simulink model "EHB_MOTOR0313"  (R2022a)
settings: Solver=FixedStepAuto  StartTime=0.0  StopTime=10  FixedStep=0.0001  RelTol=1e-3  EnableMultiTasking=on
undefined symbols (not defined in the file): Cos_Table, Cos_Table1, Sin_BreakPoint, Sin_BreakPoint1, Sin_Table, Sin_Table1
libraries: simulink x7
(part 1 of 2)
settings Model: Creator=dell  LastModifiedBy=12399
settings SolverCC: AlgebraicLoopSolver=TrustRegion  PositivePriorityOrder=on  AutoInsertRateTranBlk=on
settings DataIOCC: LimitDataPoints=on  SaveFormat=Structure  SignalLoggingSaveFormat=ModelDataLogs  ReturnWorkspaceOutputs=off
settings OptimizationCC: DefaultParameterBehavior=Inlined  UseDivisionForNetSlopeComputation=on  InlineInvariantSignals=on  ExpressionDepthLimit=2147483647  ZeroExternalMemoryAtStartup=off  NoFixptDivByZeroProtection=on  EfficientFloat2IntCast=on  LifeSpan=1  MaxStackSize=64  EfficientTunableParamExpr=on
settings DebuggingCC: CheckSSInitialOutputMsg=off  UnderspecifiedInitializationDetection=Classic  MergeDetectMultiDrivingBlocksExec=none  SignalResolutionControl=TryResolveAll  SolverPrmCheckMsg=warning  ParameterOverflowMsg=none  ParameterPrecisionLossMsg=none  FcnCallInpInsideContextMsg=warning  UnconnectedInputMsg=warning  UnconnectedOutputMsg=warning  UnconnectedLineMsg=warning  AssertControl=EnableAll  StateNameClashWarn=warning  SFUnexpectedBacktrackingDiag=warning  SFNoUnconditionalDefaultTransitionDiag=warning  SFExecutionAtInitializationDiag=none  SFMachineParentedDataDiag=warning  ArithmeticOperatorsInVariantConditions=warning
settings HardwareCC: ProdBitPerPointer=32  ProdBitPerSizeT=32  ProdBitPerPtrDiffT=32  ProdLargestAtomicInteger=Integer  ProdLargestAtomicFloat=None  ProdIntDivRoundTo=Undefined  ProdEndianess=Unspecified  ProdWordSize=32  ProdHWDeviceType=Generic->32-bit Embedded Processor  TargetBitPerPointer=64  TargetBitPerSizeT=64  TargetBitPerPtrDiffT=64  TargetLargestAtomicInteger=Integer  TargetLongLongMode=on  TargetIntDivRoundTo=Zero  TargetEndianess=LittleEndian  TargetWordSize=64  TargetHWDeviceType=MATLAB Host  ProdEqTarget=off
settings ModelReferenceCC: UpdateModelReferenceTargets=IfOutOfDate  PropagateSignalLabelsOutOfModel=off
settings SFSimCC: SimUseLocalCustomCode=off  MATLABDynamicMemAlloc=off  CustomCodeUndefinedFunction=UseInterfaceOnly
settings SFSimCC: SimCustomHeaderCode=|
  | #define MCU_IDLE_ST     0
  | #define MCU_INIT_ST     1
  | #define MCU_START_ST    2
  | #define MCU_RUN_ST      3
  | #define MCU_FAULT_ST    4
  | #define MCU_WAIT_ST     5
  | 
  | // MCU_IDLE_ST = 0;
  | // MCU_INIT_ST = 1;
  | // MCU_START_ST = 2;
  | // MCU_RUN_ST = 3;
  | // MCU_FAULT_ST = 4;
  | // MCU_WAIT_ST = 5;
settings RTWCC: SystemTargetFile=ert.tlc  TemplateMakefile=ert_default_tmf  RTWUseLocalCustomCode=off  RTWUseSimCustomCode=on  IncludeHyperlinkInReport=on
settings RTWCC: CustomHeaderCode=|
  | #define MCU_IDLE_ST     0
  | #define MCU_INIT_ST     1
  | #define MCU_START_ST    2
  | #define MCU_RUN_ST      3
  | #define MCU_FAULT_ST    4
  | #define MCU_WAIT_ST     5
  | 
  | // MCU_IDLE_ST = 0;
  | // MCU_INIT_ST = 1;
  | // MCU_START_ST = 2;
  | // MCU_RUN_ST = 3;
  | // MCU_FAULT_ST = 4;
  | // MCU_WAIT_ST = 5;
settings CodeAppCC: GenerateComments=off  IgnoreCustomStorageClasses=off  CustomSymbolStrType=$N$R$M  SimulinkBlockComments=off  MATLABSourceComments=on  InternalIdentifier=Classic
settings ERTTargetCC: MultiwordLength=2048  IncludeFileDelimiter=UseQuote  SupportContinuousTime=on  InlinedParameterPlacement=NonHierarchical  ERTCustomFileTemplate=example_file_process.tlc  GlobalDataDefinition=InSeparateSourceFile  DataDefinitionFile=EHB_MOTOR_data.c  GlobalDataReference=InSeparateHeaderFile  ERTFilePackagingFormat=CompactWithDataFile  DataReferenceFile=EHB_MOTOR.h  ConvertIfToSwitch=off  SuppressUnreachableDefaultCases=off  IndentStyle=Allman  IndentSize=4  MemSecPackage=mpt
settings ConfigComp: CovMetricSettings=dw  CovSaveCumulativeToWorkspaceVar=on  CovSaveSingleToWorkspaceVar=on  CovExternalEMLEnable=off  CovSFcnEnable=off
settings SimscapeCC: SimscapeNormalizeSystem=off
settings ConfigurationSet: Description=SimMechanics 2G

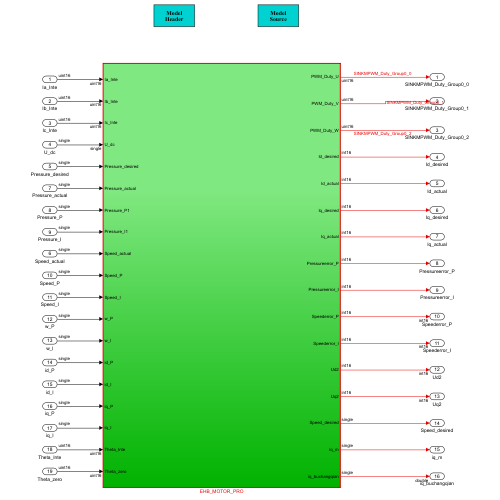
[thumbnail: Simulink's stored preview of the top-level diagram]
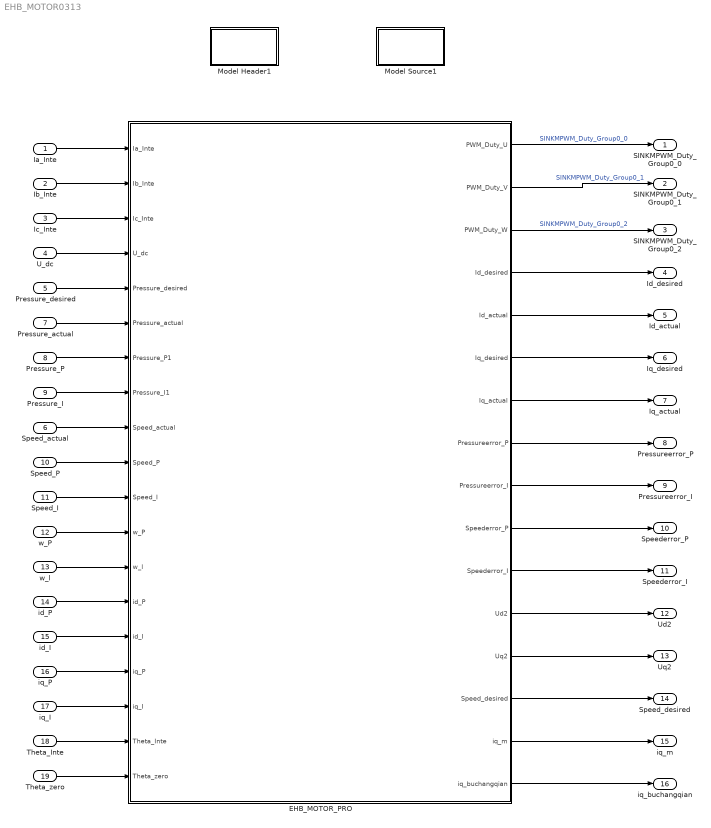
== system EHB_MOTOR0313 ==
  Ia_Inte : Inport  OutDataTypeStr=uint16
  Ib_Inte : Inport  Port=2  OutDataTypeStr=uint16
  Ic_Inte : Inport  Port=3  OutDataTypeStr=uint16
  U_dc : Inport  Port=4  OutDataTypeStr=single
  Pressure_desired : Inport  Port=5  OutDataTypeStr=single
  Speed_actual : Inport  Port=6  OutDataTypeStr=single
  Pressure_actual : Inport  Port=7  OutDataTypeStr=single
  Pressure_P : Inport  Port=8  OutDataTypeStr=single
  Pressure_I : Inport  Port=9  OutDataTypeStr=single
  Speed_P : Inport  Port=10  OutDataTypeStr=single
  Speed_I : Inport  Port=11  OutDataTypeStr=single
  w_P : Inport  Port=12  OutDataTypeStr=single
  w_l : Inport  Port=13  OutDataTypeStr=single
  id_P : Inport  Port=14  OutDataTypeStr=single
  id_I : Inport  Port=15  OutDataTypeStr=single
  iq_P : Inport  Port=16  OutDataTypeStr=single
  iq_I : Inport  Port=17  OutDataTypeStr=single
  Theta_Inte : Inport  Port=18  OutDataTypeStr=uint16
  Theta_zero : Inport  Port=19  OutDataTypeStr=uint16
  EHB_MOTOR_PRO : Subsystem  TreatAsAtomicUnit=on  RTWFcnName=isr_can_rx
      settings: MinAlgLoopOccurrences=on
  Model Header1 : Subsystem  mask(Model Header){ShowInLibBrowser=0}
      mask prompts: ShowInLibBrowser "Simulink:masks:CustCodeMaskParam1_MP"
      settings: CopyFcn=cccopyfcn(gcb)  OpenFcn=ccopenfcn('Model Header')
      mask Help: eval('feval(''rtwprivate'',''rtwhelpview'',''rtw_model_header_block'')');
      mask Display: disp('Model\nHeader');
  Model Source1 : Subsystem  mask(Model Source){ShowInLibBrowser=0}
      mask prompts: ShowInLibBrowser "Simulink:masks:CustCodeMaskParam1_MP"
      settings: CopyFcn=cccopyfcn(gcb)  OpenFcn=ccopenfcn('Model Source')
      mask Help: eval('feval(''rtwprivate'',''rtwhelpview'',''rtw_model_source_block'')');
      mask Display: disp('Model\nSource');
  SINKMPWM_Duty_Group0_0 : Outport  VectorParamsAs1DForOutWhenUnconnected=off
  SINKMPWM_Duty_Group0_1 : Outport  Port=2  VectorParamsAs1DForOutWhenUnconnected=off
  SINKMPWM_Duty_Group0_2 : Outport  Port=3  VectorParamsAs1DForOutWhenUnconnected=off
  Id_desired : Outport  Port=4  VectorParamsAs1DForOutWhenUnconnected=off
  Id_actual : Outport  Port=5  VectorParamsAs1DForOutWhenUnconnected=off
  Iq_desired : Outport  Port=6  VectorParamsAs1DForOutWhenUnconnected=off
  Iq_actual : Outport  Port=7  VectorParamsAs1DForOutWhenUnconnected=off
  Pressureerror_P : Outport  Port=8  VectorParamsAs1DForOutWhenUnconnected=off
  Pressureerror_I : Outport  Port=9  VectorParamsAs1DForOutWhenUnconnected=off
  Speederror_P : Outport  Port=10  OutDataTypeStr=int16  VectorParamsAs1DForOutWhenUnconnected=off
  Speederror_I : Outport  Port=11  OutDataTypeStr=int16  VectorParamsAs1DForOutWhenUnconnected=off
  Ud2 : Outport  Port=12  OutDataTypeStr=int16  VectorParamsAs1DForOutWhenUnconnected=off
  Uq2 : Outport  Port=13  OutDataTypeStr=int16  VectorParamsAs1DForOutWhenUnconnected=off
  Speed_desired : Outport  Port=14
  iq_m : Outport  Port=15
  iq_buchangqian : Outport  Port=16
  wires:
  EHB_MOTOR_PRO/1(PWM_Duty_U) -> SINKMPWM_Duty_Group0_0/1  "SINKMPWM_Duty_Group0_0"
  EHB_MOTOR_PRO/2(PWM_Duty_V) -> SINKMPWM_Duty_Group0_1/1  "SINKMPWM_Duty_Group0_1"
  EHB_MOTOR_PRO/3(PWM_Duty_W) -> SINKMPWM_Duty_Group0_2/1  "SINKMPWM_Duty_Group0_2"
  Theta_Inte/1 -> EHB_MOTOR_PRO/18(Theta_Inte)
  Ia_Inte/1 -> EHB_MOTOR_PRO/1(Ia_Inte)
  U_dc/1 -> EHB_MOTOR_PRO/4(U_dc)
  Ib_Inte/1 -> EHB_MOTOR_PRO/2(Ib_Inte)
  id_P/1 -> EHB_MOTOR_PRO/14(id_P)
  id_I/1 -> EHB_MOTOR_PRO/15(id_I)
  iq_P/1 -> EHB_MOTOR_PRO/16(iq_P)
  iq_I/1 -> EHB_MOTOR_PRO/17(iq_I)
  Theta_zero/1 -> EHB_MOTOR_PRO/19(Theta_zero)
  Pressure_desired/1 -> EHB_MOTOR_PRO/5(Pressure_desired)
  Speed_actual/1 -> EHB_MOTOR_PRO/9(Speed_actual)
  Speed_P/1 -> EHB_MOTOR_PRO/10(Speed_P)
  Speed_I/1 -> EHB_MOTOR_PRO/11(Speed_I)
  EHB_MOTOR_PRO/5(Id_actual) -> Id_actual/1
  EHB_MOTOR_PRO/6(Iq_desired) -> Iq_desired/1
  EHB_MOTOR_PRO/7(Iq_actual) -> Iq_actual/1
  w_l/1 -> EHB_MOTOR_PRO/13(w_l)
  EHB_MOTOR_PRO/10(Speederror_P) -> Speederror_P/1
  EHB_MOTOR_PRO/11(Speederror_I) -> Speederror_I/1
  EHB_MOTOR_PRO/4(Id_desired) -> Id_desired/1
  Ic_Inte/1 -> EHB_MOTOR_PRO/3(Ic_Inte)
  EHB_MOTOR_PRO/12(Ud2) -> Ud2/1
  EHB_MOTOR_PRO/13(Uq2) -> Uq2/1
  Pressure_actual/1 -> EHB_MOTOR_PRO/6(Pressure_actual)
  Pressure_I/1 -> EHB_MOTOR_PRO/8(Pressure_I1)
  Pressure_P/1 -> EHB_MOTOR_PRO/7(Pressure_P1)
  EHB_MOTOR_PRO/8(Pressureerror_P) -> Pressureerror_P/1
  EHB_MOTOR_PRO/9(Pressureerror_I) -> Pressureerror_I/1
  EHB_MOTOR_PRO/14(Speed_desired) -> Speed_desired/1
  w_P/1 -> EHB_MOTOR_PRO/12(w_P)
  EHB_MOTOR_PRO/15(iq_m) -> iq_m/1
  EHB_MOTOR_PRO/16(iq_buchangqian) -> iq_buchangqian/1

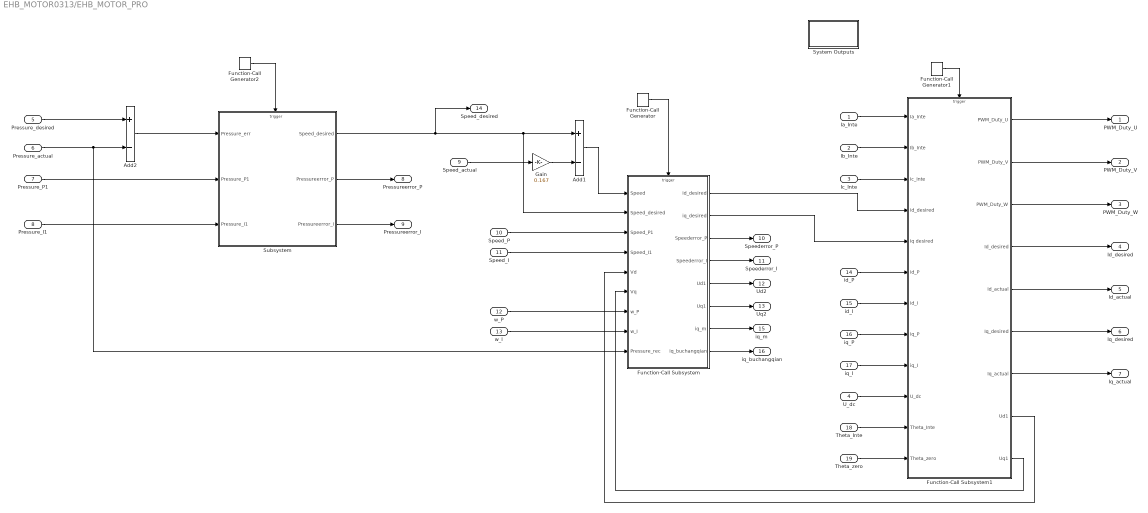
== system EHB_MOTOR0313/EHB_MOTOR_PRO ==
  Ia_Inte : Inport  OutDataTypeStr=uint16
  Ib_Inte : Inport  Port=2  OutDataTypeStr=uint16
  Ic_Inte : Inport  Port=3  OutDataTypeStr=uint16
  U_dc : Inport  Port=4  OutDataTypeStr=single
  Pressure_desired : Inport  Port=5
  Pressure_actual : Inport  Port=6
  Pressure_P1 : Inport  Port=7
  Pressure_I1 : Inport  Port=8
  Speed_actual : Inport  Port=9
  Speed_P : Inport  Port=10
  Speed_I : Inport  Port=11
  w_P : Inport  Port=12
  w_l : Inport  Port=13
  id_P : Inport  Port=14
  id_I : Inport  Port=15
  iq_P : Inport  Port=16
  iq_I : Inport  Port=17
  Theta_Inte : Inport  Port=18  OutDataTypeStr=uint16
  Theta_zero : Inport  Port=19  OutDataTypeStr=uint16
  Add1 : Sum  Inputs=+-  OutDataTypeStr=single
  Add2 : Sum  Inputs=+-  OutDataTypeStr=single
  Function-Call Generator : simulink/Ports & Subsystems/Function-Call Generator  sample_time=2e-3  numberOfIterations=1  DisallowWideOutput=off
  Function-Call Generator1 : simulink/Ports & Subsystems/Function-Call Generator  sample_time=1e-4  numberOfIterations=1  DisallowWideOutput=off
  Function-Call Generator2 : simulink/Ports & Subsystems/Function-Call Generator  sample_time=4e-3  numberOfIterations=1  DisallowWideOutput=off
  Function-Call Subsystem : Subsystem  TreatAsAtomicUnit=on
  Function-Call Subsystem1 : Subsystem  TreatAsAtomicUnit=on
  Gain : Gain  Gain=0.167
  Subsystem : Subsystem
  System Outputs : Subsystem  mask(System Outputs){ShowInLibBrowser=0}
      mask prompts: ShowInLibBrowser "Simulink:masks:CustCodeMaskParam1_MP"
      settings: CopyFcn=cccopyfcn(gcb)  OpenFcn=ccopenfcn('System Outputs Function')
      mask Help: eval('feval(''rtwprivate'',''rtwhelpview'',''rtw_sys_outputs_block'')');
      mask Display: disp('System\nOutputs');
  PWM_Duty_U : Outport  VectorParamsAs1DForOutWhenUnconnected=off
  PWM_Duty_V : Outport  Port=2  VectorParamsAs1DForOutWhenUnconnected=off
  PWM_Duty_W : Outport  Port=3  VectorParamsAs1DForOutWhenUnconnected=off
  Id_desired : Outport  Port=4  VectorParamsAs1DForOutWhenUnconnected=off
  Id_actual : Outport  Port=5  VectorParamsAs1DForOutWhenUnconnected=off
  Iq_desired : Outport  Port=6  VectorParamsAs1DForOutWhenUnconnected=off
  Iq_actual : Outport  Port=7  VectorParamsAs1DForOutWhenUnconnected=off
  Pressureerror_P : Outport  Port=8  OutDataTypeStr=int16  VectorParamsAs1DForOutWhenUnconnected=off
  Pressureerror_I : Outport  Port=9  OutDataTypeStr=int16  VectorParamsAs1DForOutWhenUnconnected=off
  Speederror_P : Outport  Port=10  OutDataTypeStr=int16  VectorParamsAs1DForOutWhenUnconnected=off
  Speederror_I : Outport  Port=11  OutDataTypeStr=int16  VectorParamsAs1DForOutWhenUnconnected=off
  Ud2 : Outport  Port=12  OutDataTypeStr=int16  VectorParamsAs1DForOutWhenUnconnected=off
  Uq2 : Outport  Port=13  OutDataTypeStr=int16  VectorParamsAs1DForOutWhenUnconnected=off
  Speed_desired : Outport  Port=14
  iq_m : Outport  Port=15  OutDataTypeStr=single  VectorParamsAs1DForOutWhenUnconnected=off
  iq_buchangqian : Outport  Port=16  OutDataTypeStr=single  VectorParamsAs1DForOutWhenUnconnected=off
  wires:
  Speed_actual/1 -> Gain/1
  Gain/1 -> Add1/2
  Ia_Inte/1 -> Function-Call Subsystem1/1(Ia_Inte)
  Ib_Inte/1 -> Function-Call Subsystem1/2(Ib_Inte)
  Function-Call Subsystem/1(id_desired) -> Function-Call Subsystem1/4(id_desired)
  id_P/1 -> Function-Call Subsystem1/6(id_P)
  id_I/1 -> Function-Call Subsystem1/7(id_I)
  iq_P/1 -> Function-Call Subsystem1/8(iq_P)
  iq_I/1 -> Function-Call Subsystem1/9(iq_I)
  U_dc/1 -> Function-Call Subsystem1/10(U_dc)
  Theta_Inte/1 -> Function-Call Subsystem1/11(Theta_Inte)
  Theta_zero/1 -> Function-Call Subsystem1/12(Theta_zero)
  Function-Call Subsystem1/1(PWM_Duty_U) -> PWM_Duty_U/1
  Function-Call Subsystem1/2(PWM_Duty_V) -> PWM_Duty_V/1
  Function-Call Subsystem1/3(PWM_Duty_W) -> PWM_Duty_W/1
  Add1/1 -> Function-Call Subsystem/1(Speed)
  Speed_P/1 -> Function-Call Subsystem/3(Speed_P1)
  Speed_I/1 -> Function-Call Subsystem/4(Speed_I1)
  Function-Call Generator/1 -> Function-Call Subsystem/Trigger
  Function-Call Generator1/1 -> Function-Call Subsystem1/Trigger
  Function-Call Subsystem1/5(Id_actual) -> Id_actual/1
  Function-Call Subsystem1/6(Iq_desired) -> Iq_desired/1
  Function-Call Subsystem1/7(Iq_actual) -> Iq_actual/1
  Function-Call Subsystem1/8(Ud1) -> Function-Call Subsystem/5(Vd)
  Function-Call Subsystem1/9(Uq1) -> Function-Call Subsystem/6(Vq)
  Function-Call Subsystem1/4(Id_desired) -> Id_desired/1
  Function-Call Subsystem/3(Speederror_P) -> Speederror_P/1
  Function-Call Subsystem/4(Speederror_I) -> Speederror_I/1
  Ic_Inte/1 -> Function-Call Subsystem1/3(Ic_Inte)
  w_l/1 -> Function-Call Subsystem/8(w_I)
  Function-Call Subsystem/5(Ud1) -> Ud2/1
  Function-Call Subsystem/6(Uq1) -> Uq2/1
  Pressure_desired/1 -> Add2/1
  Pressure_I1/1 -> Subsystem/3(Pressure_I1)
  Pressure_P1/1 -> Subsystem/2(Pressure_P1)
  Add2/1 -> Subsystem/1(Pressure_err)
  Subsystem/3(Pressureerror_I) -> Pressureerror_I/1
  Subsystem/2(Pressureerror_P) -> Pressureerror_P/1
  Function-Call Generator2/1 -> Subsystem/Trigger
  Subsystem/1(Speed_desired) -> Speed_desired/1, Function-Call Subsystem/2(Speed_desired), Add1/1
  w_P/1 -> Function-Call Subsystem/7(w_P)
  Function-Call Subsystem/2(iq_desired) -> Function-Call Subsystem1/5(Iq desired)
  Function-Call Subsystem/7(iq_m) -> iq_m/1
  Function-Call Subsystem/8(iq_buchangqian) -> iq_buchangqian/1
  Pressure_actual/1 -> Function-Call Subsystem/9(Pressure_rec), Add2/2

== system EHB_MOTOR0313/Model Header1 ==

== system EHB_MOTOR0313/Model Source1 ==

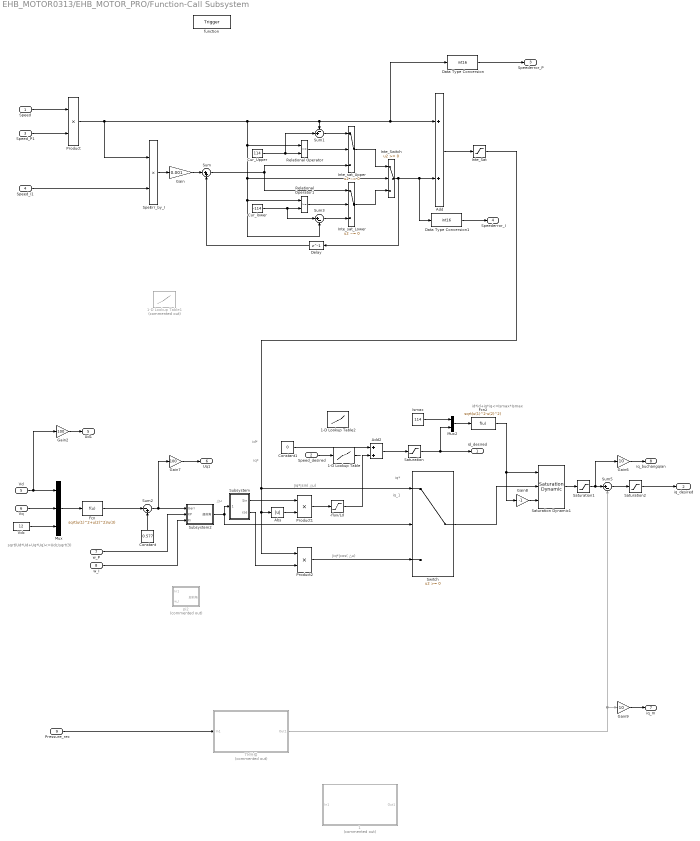
== system EHB_MOTOR0313/EHB_MOTOR_PRO/Function-Call Subsystem ==
  note: iq*
  note: id*
  note: |iq*|cos( △u)
  note: iq*
  note: iq_1
  note: sqrt(Ud*Ud+Uq*Uq)<=Udc/sqrt(3)
  note: |iq*|sin( △u)
  note: id*id+iq*iq<=Ismax*Ismax
  note: △u
  Speed : Inport
  Speed_desired : Inport  Port=2
  Speed_P1 : Inport  Port=3
  Speed_I1 : Inport  Port=4
  Vd : Inport  Port=5  OutDataTypeStr=single
  Vq : Inport  Port=6  OutDataTypeStr=single
  w_P : Inport  Port=7  OutDataTypeStr=single
  w_I : Inport  Port=8  OutDataTypeStr=single
  Pressure_rec : Inport  Port=9
  function : TriggerPort  TriggerType=function-call  VariantControl=(inherit)
  -flux/Ld : Saturate  UpperLimit=0  LowerLimit=-76
  1 : Subsystem  Commented=on
  1-D Lookup Table : Lookup_n-D  NumberOfTableDimensions=1  BreakpointsForDimension1=[0;2200;2345;2347;2348;2351;2355;2383;2386;2420;2421;2537;2654;2812;3000]  Table=[0;-0.002;-0.07;-0.1;-0.2;-0.3;-0.5;-1;-2;-4;-5;-9;-16;-18;-24]  InternalRulePriority=Speed  RndMeth=Simplest
  1-D Lookup Table1 : Lookup_n-D  Commented=on  NumberOfTableDimensions=1  BreakpointsForDimension1=[0;2345;2347;2348;2351;2355;2383;2386;2420;2421;2537;2654;2812;3000]  Table=[0;-0.002;-0.007;-0.025;-0.117;-0.293;-0.79;-1.08;-2.944;-3.234;-7.193;-12.183;-16.24;-20]  InternalRulePriority=Speed  RndMeth=Simplest
  1-D Lookup Table2 : Lookup_n-D  NumberOfTableDimensions=1  BreakpointsForDimension1=[0;2200;2345;2347;2348;2351;2355;2383;2386;2420;2421;2537;2654;2812;3000]  Table=[0;-0.002;-0.07;-0.1;-0.2;-0.3;-0.5;-1;-2;-4;-5;-9;-16;-18;-24]  InternalRulePriority=Speed  RndMeth=Simplest
  Abs : Abs  SaturateOnIntegerOverflow=off
  Add : Sum  OutDataTypeStr=single
  Add2 : Sum  AccumDataTypeStr=single  OutDataTypeStr=single
  Constant : Constant  Value=0.577  OutDataTypeStr=single
  Constant1 : Constant  Value=0  OutDataTypeStr=single
  Cur_Upper : Constant  Value=114  OutDataTypeStr=single
  Cur_lower : Constant  Value=-114  OutDataTypeStr=single
  Data Type Conversion : DataTypeConversion  OutDataTypeStr=int16  SaturateOnIntegerOverflow=off  RndMeth=Floor
  Data Type Conversion1 : DataTypeConversion  OutDataTypeStr=int16  SaturateOnIntegerOverflow=off  RndMeth=Floor
  Delay : Delay  DelayLength=1
  Fcn : Fcn  Expr=sqrt(u(1)^2+u(2)^2)/u(3)
  Fcn2 : Fcn  Expr=sqrt(u(1)^2-u(2)^2)
  Gain : Gain  Gain=0.001
  Gain2 : Gain  Gain=100  ParamDataTypeStr=int16  OutDataTypeStr=int16
  Gain6 : Gain  Gain=10
  Gain7 : Gain  Gain=100  ParamDataTypeStr=int16  OutDataTypeStr=int16
  Gain8 : Gain  Gain=-1
  Gain9 : Gain  Gain=10
  Inte_Sat : Saturate  UpperLimit=114  LowerLimit=-114
  Inte_Switch : Switch  SaturateOnIntegerOverflow=off  InputSameDT=off
  Inte_sat_Lower : Switch  Criteria=u2 ~= 0  OutDataTypeStr=single  SaturateOnIntegerOverflow=off  InputSameDT=off
  Inte_sat_Upper : Switch  Criteria=u2 ~= 0  OutDataTypeStr=single  SaturateOnIntegerOverflow=off  InputSameDT=off
  Ismax : Constant  Value=114  OutDataTypeStr=single  SampleTime=-1
  Mux : Mux  Inputs=3
  Mux2 : Mux  Inputs=2
  Product : Product  OutDataTypeStr=single
  Product1 : Product  RndMeth=Zero
  Product2 : Product  RndMeth=Zero
  Relational Operator : RelationalOperator  OutDataTypeStr=boolean  RndMeth=Simplest  InputSameDT=off
  Relational Operator1 : RelationalOperator  OutDataTypeStr=boolean  RndMeth=Simplest  InputSameDT=off
  Saturation : Saturate  UpperLimit=100  LowerLimit=-100  OutDataTypeStr=single
  Saturation Dynamic1 : simulink/Discontinuities/Saturation Dynamic  OutMin=[]  OutMax=[]  OutDataTypeStr=Inherit: Same as second input  OutDataType=fixdt(1, 16)  OutScaling=2^-10  DoSatur=off
  Saturation1 : Saturate  UpperLimit=114  LowerLimit=-114
  Saturation2 : Saturate  UpperLimit=114  LowerLimit=-114
  SpeErr_by_I : Product  OutDataTypeStr=single
  Subsystem : Subsystem
  Subsystem2 : Subsystem
  Sum : Sum  Inputs=|++
  Sum1 : Sum  Inputs=-+|  OutDataTypeStr=single
  Sum2 : Sum  Inputs=|-+
  Sum3 : Sum  Inputs=|+-  OutDataTypeStr=single
  Sum5 : Sum  Inputs=|+-
  Switch : Switch  SaturateOnIntegerOverflow=off  InputSameDT=off
  TM补偿 : Subsystem  Commented=on
  Vdc : Constant  Value=12  OutDataTypeStr=single
  pi2 : Subsystem  Commented=on
  id_desired : Outport
  iq_desired : Outport  Port=2
  Speederror_P : Outport  Port=3  OutDataTypeStr=int16  VectorParamsAs1DForOutWhenUnconnected=off
  Speederror_I : Outport  Port=4  OutDataTypeStr=int16  VectorParamsAs1DForOutWhenUnconnected=off
  Ud1 : Outport  Port=5  OutDataTypeStr=int16  VectorParamsAs1DForOutWhenUnconnected=off
  Uq1 : Outport  Port=6  OutDataTypeStr=int16  VectorParamsAs1DForOutWhenUnconnected=off
  iq_m : Outport  Port=7
  iq_buchangqian : Outport  Port=8
  wires:
  Relational Operator/1 -> Inte_sat_Upper/2
  Inte_sat_Upper/1 -> Inte_Switch/1
  Speed_I1/1 -> SpeErr_by_I/2
  Speed_P1/1 -> Product/2
  Delay/1 -> Sum/2
  Sum1/1 -> Inte_sat_Upper/1
  Relational Operator1/1 -> Inte_sat_Lower/2
  Cur_Upper/1 -> Sum1/2, Relational Operator/2
  Sum3/1 -> Inte_sat_Lower/3
  SpeErr_by_I/1 -> Gain/1
  Inte_sat_Lower/1 -> Inte_Switch/3
  Speed/1 -> Product/1
  Add/1 -> Inte_Sat/1
  Sum/1 -> Inte_sat_Upper/3, Inte_sat_Lower/1
  Cur_lower/1 -> Sum3/1, Relational Operator1/2
  Gain/1 -> Sum/1
  Abs/1 -> Product1/2
  Constant/1 -> Sum2/2
  Vd/1 -> Gain2/1, Mux/1
  Subsystem/1(Sin) -> Product1/1
  Product2/1 -> Switch/3
  Add2/1 -> Saturation/1
  Ismax/1 -> Mux2/1
  Subsystem2/1(超前角) -> Subsystem/1(超前角), Switch/2
  Mux/1 -> Fcn/1
  w_I/1 -> Subsystem2/3(Ki)
  Inte_Sat/1 -> Product2/1, Abs/1, Switch/1
  Sum2/1 -> Subsystem2/1(Uerr), Gain7/1
  Switch/1 -> Saturation Dynamic1/2
  Vq/1 -> Mux/2
  Product1/1 -> -flux/Ld/1
  Gain7/1 -> Uq1/1
  Subsystem/2(cos) -> Product2/2
  Constant1/1 -> Add2/1
  Gain2/1 -> Ud1/1
  Fcn2/1 -> Gain8/1, Saturation Dynamic1/1
  Saturation/1 -> Mux2/2, id_desired/1
  Mux2/1 -> Fcn2/1
  Saturation Dynamic1/1 -> Saturation1/1
  Fcn/1 -> Sum2/1
  Gain8/1 -> Saturation Dynamic1/3
  1-D Lookup Table/1 -> ?
  -flux/Ld/1 -> Add2/2
  Speed_desired/1 -> 1-D Lookup Table/1
  w_P/1 -> Subsystem2/2(KP)
  Product/1 -> Sum1/1, Data Type Conversion/1, Add/1, Inte_Switch/2, Sum3/2, Relational Operator1/1, Relational Operator/1, SpeErr_by_I/1
  Inte_Switch/1 -> Data Type Conversion1/1, Add/2, Delay/1
  Data Type Conversion/1 -> Speederror_P/1
  Data Type Conversion1/1 -> Speederror_I/1
  Vdc/1 -> Mux/3
  Saturation2/1 -> iq_desired/1
  Gain9/1 -> iq_m/1
  Sum5/1 -> Saturation2/1
  Saturation1/1 -> Gain6/1, Sum5/1
  Gain6/1 -> iq_buchangqian/1
  TM补偿/1(Out1) -> Gain9/1, Sum5/2
  Pressure_rec/1 -> TM补偿/1(In1)

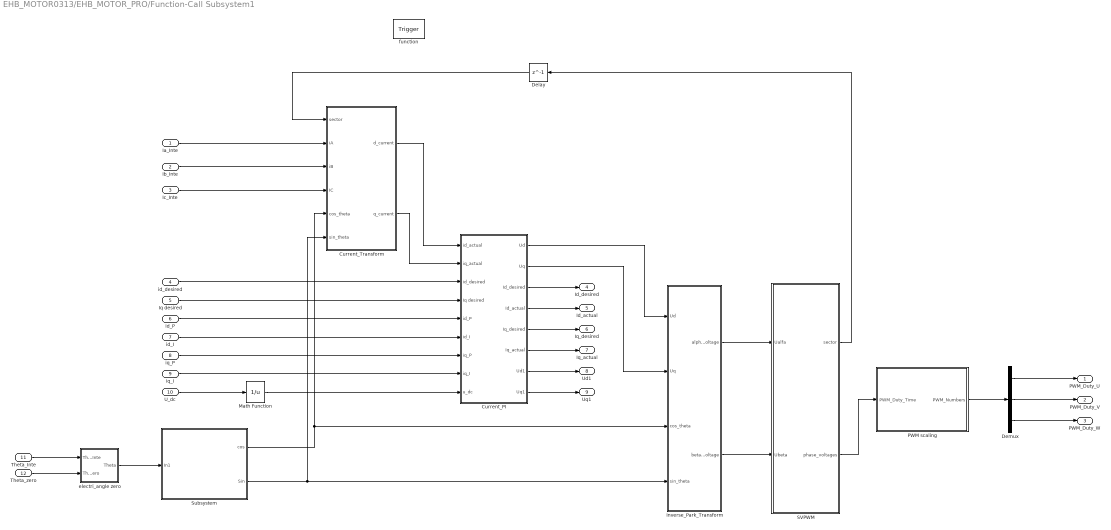
== system EHB_MOTOR0313/EHB_MOTOR_PRO/Function-Call Subsystem1 ==
  Ia_Inte : Inport  OutDataTypeStr=uint16
  Ib_Inte : Inport  Port=2  OutDataTypeStr=uint16
  Ic_Inte : Inport  Port=3  OutDataTypeStr=uint16
  id_desired : Inport  Port=4  OutDataTypeStr=single
  Iq desired : Inport  Port=5  OutDataTypeStr=single
  id_P : Inport  Port=6
  id_I : Inport  Port=7
  iq_P : Inport  Port=8
  iq_I : Inport  Port=9
  U_dc : Inport  Port=10  OutDataTypeStr=single
  Theta_Inte : Inport  Port=11  OutDataTypeStr=uint16
  Theta_zero : Inport  Port=12  OutDataTypeStr=uint16
  function : TriggerPort  TriggerType=function-call  VariantControl=(inherit)
  Current_PI : Subsystem
  Current_Transform : Subsystem
  Delay : Delay  DelayLength=1
  Demux : Demux  Outputs=3
  Inverse_Park_Transform : Subsystem
  Math Function : Math  Operator=reciprocal  SignedPower=on  OutDataTypeStr=single
  PWM scaling : Subsystem
  SVPWM : Subsystem
  Subsystem : Subsystem
  electri_angle zero : Subsystem
  PWM_Duty_U : Outport  VectorParamsAs1DForOutWhenUnconnected=off
  PWM_Duty_V : Outport  Port=2  VectorParamsAs1DForOutWhenUnconnected=off
  PWM_Duty_W : Outport  Port=3  VectorParamsAs1DForOutWhenUnconnected=off
  Id_desired : Outport  Port=4  VectorParamsAs1DForOutWhenUnconnected=off
  Id_actual : Outport  Port=5  VectorParamsAs1DForOutWhenUnconnected=off
  Iq_desired : Outport  Port=6  VectorParamsAs1DForOutWhenUnconnected=off
  Iq_actual : Outport  Port=7  VectorParamsAs1DForOutWhenUnconnected=off
  Ud1 : Outport  Port=8  OutDataTypeStr=single  VectorParamsAs1DForOutWhenUnconnected=off
  Uq1 : Outport  Port=9  OutDataTypeStr=single  VectorParamsAs1DForOutWhenUnconnected=off
  wires:
  Demux/2 -> PWM_Duty_V/1
  U_dc/1 -> Math Function/1
  Demux/3 -> PWM_Duty_W/1
  id_I/1 -> Current_PI/6(id_I)
  Theta_Inte/1 -> electri_angle zero/1(Theta_Inte)
  id_P/1 -> Current_PI/5(id_P)
  Theta_zero/1 -> electri_angle zero/2(Theta_zero)
  iq_I/1 -> Current_PI/8(iq_I)
  PWM scaling/1(PWM_Numbers) -> Demux/1
  electri_angle zero/1(Theta) -> Subsystem/1(In1)
  Inverse_Park_Transform/1(alpha_voltage) -> SVPWM/1(Ualfa)
  Subsystem/2(Sin) -> Inverse_Park_Transform/4(sin_theta), Current_Transform/6(sin_theta)
  Iq desired/1 -> Current_PI/4(Iq desired)
  id_desired/1 -> Current_PI/3(id_desired)
  SVPWM/2(phase_voltages) -> PWM scaling/1(PWM_Duty_Time)
  Math Function/1 -> Current_PI/9(u_dc)
  Demux/1 -> PWM_Duty_U/1
  iq_P/1 -> Current_PI/7(iq_P)
  Current_PI/1(Ud) -> Inverse_Park_Transform/1(Ud)
  Inverse_Park_Transform/2(beta_voltage) -> SVPWM/2(Ubeta)
  Current_Transform/1(d_current) -> Current_PI/1(id_actual)
  Current_Transform/2(q_current) -> Current_PI/2(iq_actual)
  Current_PI/2(Uq) -> Inverse_Park_Transform/2(Uq)
  Subsystem/1(cos) -> Inverse_Park_Transform/3(cos_theta), Current_Transform/5(cos_theta)
  Current_PI/4(Id_actual) -> Id_actual/1
  Current_PI/5(Iq_desired) -> Iq_desired/1
  Current_PI/6(Iq_actual) -> Iq_actual/1
  Current_PI/3(Id_desired) -> Id_desired/1
  Ia_Inte/1 -> Current_Transform/2(iA)
  Ib_Inte/1 -> Current_Transform/3(iB)
  Ic_Inte/1 -> Current_Transform/4(IC)
  SVPWM/1(sector) -> Delay/1
  Delay/1 -> Current_Transform/1(sector)
  Current_PI/7(Ud1) -> Ud1/1
  Current_PI/8(Uq1) -> Uq1/1

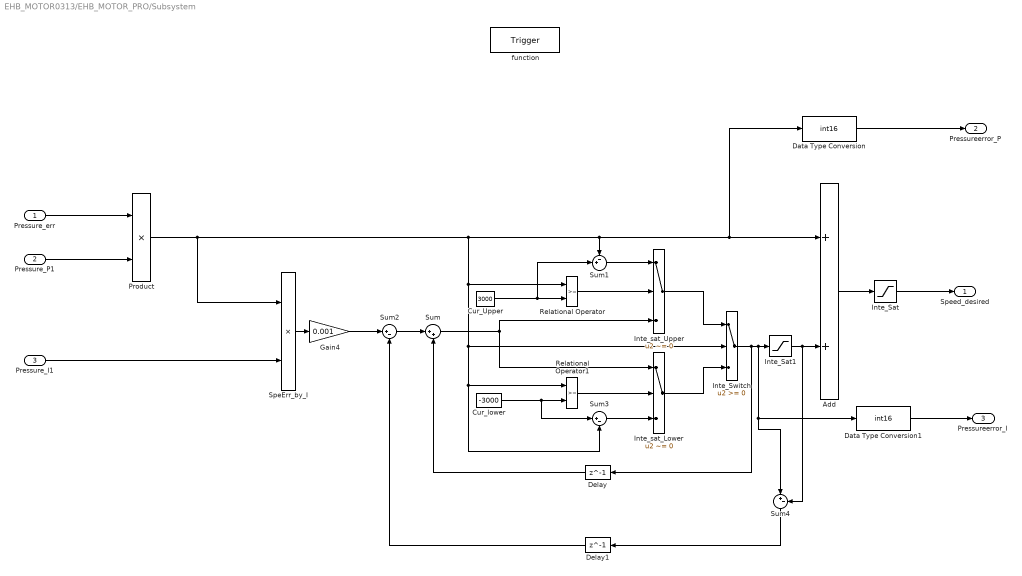
== system EHB_MOTOR0313/EHB_MOTOR_PRO/Subsystem ==
  Pressure_err : Inport
  Pressure_P1 : Inport  Port=2
  Pressure_I1 : Inport  Port=3
  function : TriggerPort  TriggerType=function-call  VariantControl=(inherit)
  Add : Sum  OutDataTypeStr=single
  Cur_Upper : Constant  Value=3000  OutDataTypeStr=single
  Cur_lower : Constant  Value=-3000  OutDataTypeStr=single
  Data Type Conversion : DataTypeConversion  OutDataTypeStr=int16  SaturateOnIntegerOverflow=off  RndMeth=Floor
  Data Type Conversion1 : DataTypeConversion  OutDataTypeStr=int16  SaturateOnIntegerOverflow=off  RndMeth=Floor
  Delay : Delay  DelayLength=1
  Delay1 : Delay  DelayLength=1
  Gain4 : Gain  Gain=0.001
  Inte_Sat : Saturate  UpperLimit=3000  LowerLimit=-3000
  Inte_Sat1 : Saturate  UpperLimit=3000  LowerLimit=-3000
  Inte_Switch : Switch  SaturateOnIntegerOverflow=off  InputSameDT=off
  Inte_sat_Lower : Switch  Criteria=u2 ~= 0  OutDataTypeStr=single  SaturateOnIntegerOverflow=off  InputSameDT=off
  Inte_sat_Upper : Switch  Criteria=u2 ~= 0  OutDataTypeStr=single  SaturateOnIntegerOverflow=off  InputSameDT=off
  Product : Product  OutDataTypeStr=single
  Relational Operator : RelationalOperator  OutDataTypeStr=boolean  RndMeth=Simplest  InputSameDT=off
  Relational Operator1 : RelationalOperator  OutDataTypeStr=boolean  RndMeth=Simplest  InputSameDT=off
  SpeErr_by_I : Product  OutDataTypeStr=single
  Sum : Sum  Inputs=|++
  Sum1 : Sum  Inputs=-+|  OutDataTypeStr=single
  Sum2 : Sum  Inputs=|+-
  Sum3 : Sum  Inputs=|+-  OutDataTypeStr=single
  Sum4 : Sum  Inputs=|+-
  Speed_desired : Outport
  Pressureerror_P : Outport  Port=2  OutDataTypeStr=int16  VectorParamsAs1DForOutWhenUnconnected=off
  Pressureerror_I : Outport  Port=3  OutDataTypeStr=int16  VectorParamsAs1DForOutWhenUnconnected=off
  wires:
  Inte_Sat/1 -> Speed_desired/1
  Inte_Switch/1 -> Delay/1, Data Type Conversion1/1, Sum4/1, Inte_Sat1/1
  Product/1 -> SpeErr_by_I/1, Inte_Switch/2, Sum3/2, Relational Operator1/1, Relational Operator/1, Sum1/1, Data Type Conversion/1, Add/1
  Pressure_err/1 -> Product/1
  Pressure_P1/1 -> Product/2
  Add/1 -> Inte_Sat/1
  Pressure_I1/1 -> SpeErr_by_I/2
  SpeErr_by_I/1 -> Gain4/1
  Inte_sat_Lower/1 -> Inte_Switch/3
  Cur_Upper/1 -> Sum1/2, Relational Operator/2
  Relational Operator/1 -> Inte_sat_Upper/2
  Delay/1 -> Sum/2
  Inte_sat_Upper/1 -> Inte_Switch/1
  Sum3/1 -> Inte_sat_Lower/3
  Cur_lower/1 -> Sum3/1, Relational Operator1/2
  Gain4/1 -> Sum2/1
  Relational Operator1/1 -> Inte_sat_Lower/2
  Sum/1 -> Inte_sat_Lower/1, Inte_sat_Upper/3
  Sum1/1 -> Inte_sat_Upper/1
  Inte_Sat1/1 -> Sum4/2, Add/2
  Sum2/1 -> Sum/1
  Delay1/1 -> Sum2/2
  Sum4/1 -> Delay1/1
  Data Type Conversion/1 -> Pressureerror_P/1
  Data Type Conversion1/1 -> Pressureerror_I/1

== system EHB_MOTOR0313/EHB_MOTOR_PRO/System Outputs ==

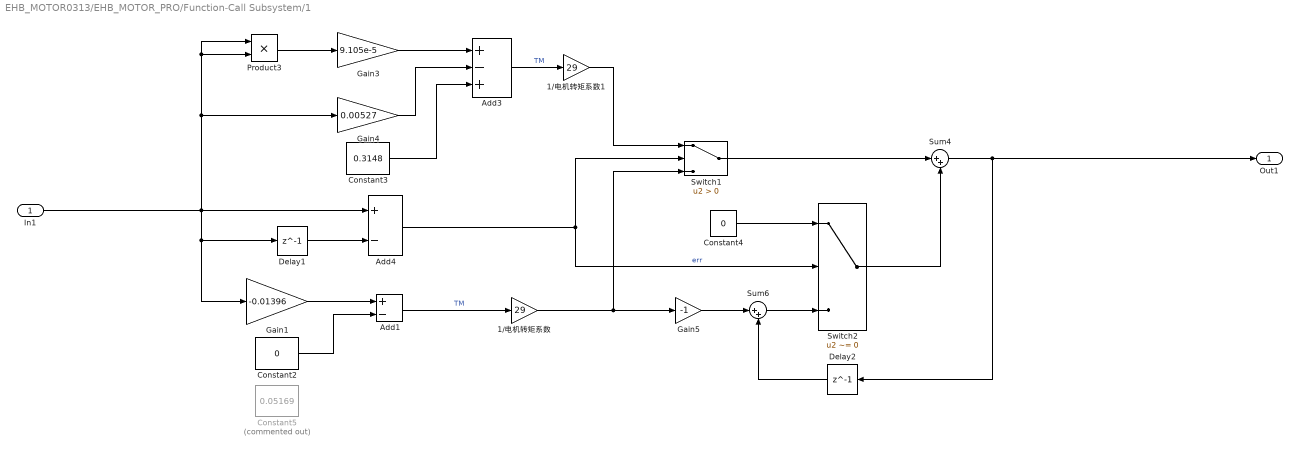
== system EHB_MOTOR0313/EHB_MOTOR_PRO/Function-Call Subsystem/1 ==
  In1 : Inport
  1/电机转矩系数 : Gain  Gain=29
  1/电机转矩系数1 : Gain  Gain=29
  Add1 : Sum  Inputs=+-
  Add3 : Sum  Inputs=+-+
  Add4 : Sum  Inputs=+-
  Constant2 : Constant  Value=0  OutDataTypeStr=single
  Constant3 : Constant  Value=0.3148  OutDataTypeStr=single
  Constant4 : Constant  Value=0  OutDataTypeStr=single
  Constant5 : Constant  Commented=on  Value=0.05169  OutDataTypeStr=single
  Delay1 : Delay  DelayLength=1
  Delay2 : Delay  DelayLength=1
  Gain1 : Gain  Gain=-0.01396
  Gain3 : Gain  Gain=9.105e-5
  Gain4 : Gain  Gain=0.00527
  Gain5 : Gain  Gain=-1
  Product3 : Product
  Sum4 : Sum  Inputs=|++
  Sum6 : Sum  Inputs=|++
  Switch1 : Switch  Criteria=u2 > Threshold  SaturateOnIntegerOverflow=off  InputSameDT=off
  Switch2 : Switch  Criteria=u2 ~= 0  SaturateOnIntegerOverflow=off  InputSameDT=off
  Out1 : Outport
  wires:
  Constant3/1 -> Add3/3
  1/电机转矩系数1/1 -> Switch1/1
  Gain5/1 -> Sum6/1
  Sum4/1 -> Delay2/1, Out1/1
  Sum6/1 -> Switch2/3
  Product3/1 -> Gain3/1
  Gain1/1 -> Add1/1
  Gain4/1 -> Add3/2
  Switch1/1 -> Sum4/1
  Switch2/1 -> Sum4/2
  Delay2/1 -> Sum6/2
  Constant4/1 -> Switch2/1
  In1/1 -> Product3/1, Product3/2, Gain4/1, Add4/1, Gain1/1, Delay1/1
  Delay1/1 -> Add4/2
  Constant2/1 -> Add1/2
  Add1/1 -> 1/电机转矩系数/1  "TM"
  Add3/1 -> 1/电机转矩系数1/1  "TM"
  Gain3/1 -> Add3/1
  Add4/1 -> Switch1/2, Switch2/2  "err"
  1/电机转矩系数/1 -> Gain5/1, Switch1/3

== system EHB_MOTOR0313/EHB_MOTOR_PRO/Function-Call Subsystem/Subsystem ==
  超前角 : Inport
  n-D Lookup Table : Lookup_n-D  NumberOfTableDimensions=1  BreakpointsForDimension1=Sin_BreakPoint1  BreakpointsForDimension3=[5, 7]  BreakpointsForDimension1DataTypeStr=Inherit: Inherit from 'Breakpoint data'  Table=Sin_Table1  TableDataTypeStr=Inherit: Inherit from 'Table data'  ExtrapMethod=Clip  InternalRulePriority=Speed  OutDataTypeStr=Inherit: Inherit from 'Table data'  RndMeth=Simplest  InputSameDT=off
  n-D Lookup Table1 : Lookup_n-D  NumberOfTableDimensions=1  BreakpointsForDimension1=Sin_BreakPoint1  BreakpointsForDimension3=[5, 7]  BreakpointsForDimension1DataTypeStr=Inherit: Inherit from 'Breakpoint data'  Table=Cos_Table1  TableDataTypeStr=Inherit: Inherit from 'Table data'  ExtrapMethod=Clip  InternalRulePriority=Speed  OutDataTypeStr=Inherit: Inherit from 'Table data'  RndMeth=Simplest  InputSameDT=off
  Sin : Outport  VectorParamsAs1DForOutWhenUnconnected=off
  cos : Outport  Port=2  VectorParamsAs1DForOutWhenUnconnected=off
  wires:
  n-D Lookup Table/1 -> Sin/1
  n-D Lookup Table1/1 -> cos/1
  超前角/1 -> n-D Lookup Table1/1, n-D Lookup Table/1

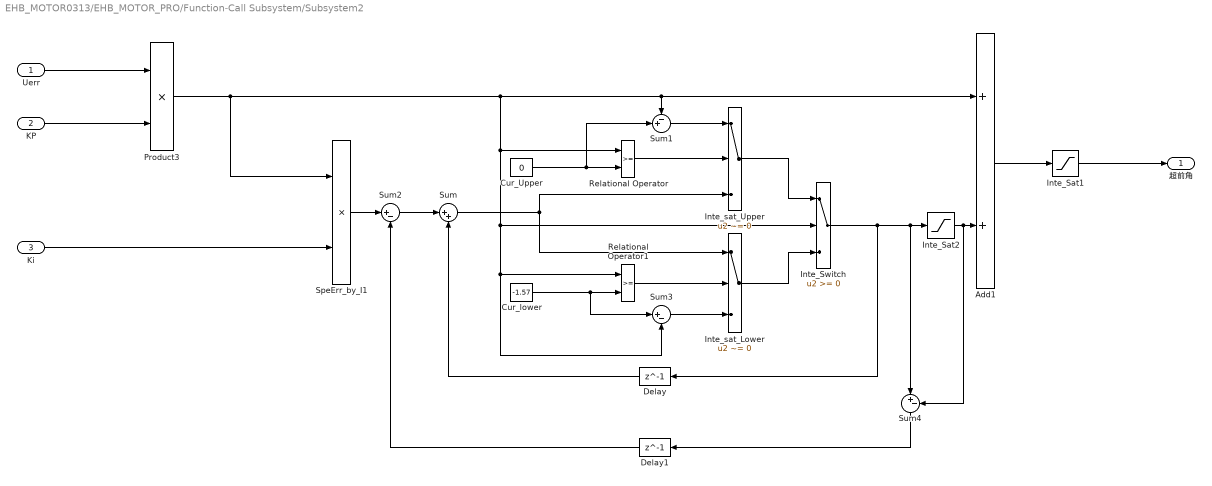
== system EHB_MOTOR0313/EHB_MOTOR_PRO/Function-Call Subsystem/Subsystem2 ==
  Uerr : Inport
  KP : Inport  Port=2
  Ki : Inport  Port=3
  Add1 : Sum  OutDataTypeStr=single
  Cur_Upper : Constant  Value=0  OutDataTypeStr=single
  Cur_lower : Constant  Value=-1.57  OutDataTypeStr=single
  Delay : Delay  DelayLength=1
  Delay1 : Delay  DelayLength=1
  Inte_Sat1 : Saturate  UpperLimit=0  LowerLimit=-1.57
  Inte_Sat2 : Saturate  UpperLimit=0  LowerLimit=-1.57
  Inte_Switch : Switch  SaturateOnIntegerOverflow=off  InputSameDT=off
  Inte_sat_Lower : Switch  Criteria=u2 ~= 0  OutDataTypeStr=single  SaturateOnIntegerOverflow=off  InputSameDT=off
  Inte_sat_Upper : Switch  Criteria=u2 ~= 0  OutDataTypeStr=single  SaturateOnIntegerOverflow=off  InputSameDT=off
  Product3 : Product  OutDataTypeStr=single
  Relational Operator : RelationalOperator  OutDataTypeStr=boolean  RndMeth=Simplest  InputSameDT=off
  Relational Operator1 : RelationalOperator  OutDataTypeStr=boolean  RndMeth=Simplest  InputSameDT=off
  SpeErr_by_I1 : Product  OutDataTypeStr=single
  Sum : Sum  Inputs=|++
  Sum1 : Sum  Inputs=-+|  OutDataTypeStr=single
  Sum2 : Sum  Inputs=|+-
  Sum3 : Sum  Inputs=|+-  OutDataTypeStr=single
  Sum4 : Sum  Inputs=|+-
  超前角 : Outport
  wires:
  Inte_Sat1/1 -> 超前角/1
  Uerr/1 -> Product3/1
  Ki/1 -> SpeErr_by_I1/2
  Add1/1 -> Inte_Sat1/1
  KP/1 -> Product3/2
  Inte_sat_Lower/1 -> Inte_Switch/3
  Cur_Upper/1 -> Sum1/2, Relational Operator/2
  Relational Operator/1 -> Inte_sat_Upper/2
  Delay/1 -> Sum/2
  Inte_sat_Upper/1 -> Inte_Switch/1
  Sum3/1 -> Inte_sat_Lower/3
  Product3/1 -> SpeErr_by_I1/1, Add1/1, Sum1/1, Inte_Switch/2, Sum3/2, Relational Operator1/1, Relational Operator/1
  Cur_lower/1 -> Sum3/1, Relational Operator1/2
  Relational Operator1/1 -> Inte_sat_Lower/2
  Sum/1 -> Inte_sat_Upper/3, Inte_sat_Lower/1
  Sum1/1 -> Inte_sat_Upper/1
  SpeErr_by_I1/1 -> Sum2/1
  Sum4/1 -> Delay1/1
  Inte_Switch/1 -> Sum4/1, Inte_Sat2/1, Delay/1
  Delay1/1 -> Sum2/2
  Sum2/1 -> Sum/1
  Inte_Sat2/1 -> Sum4/2, Add1/2

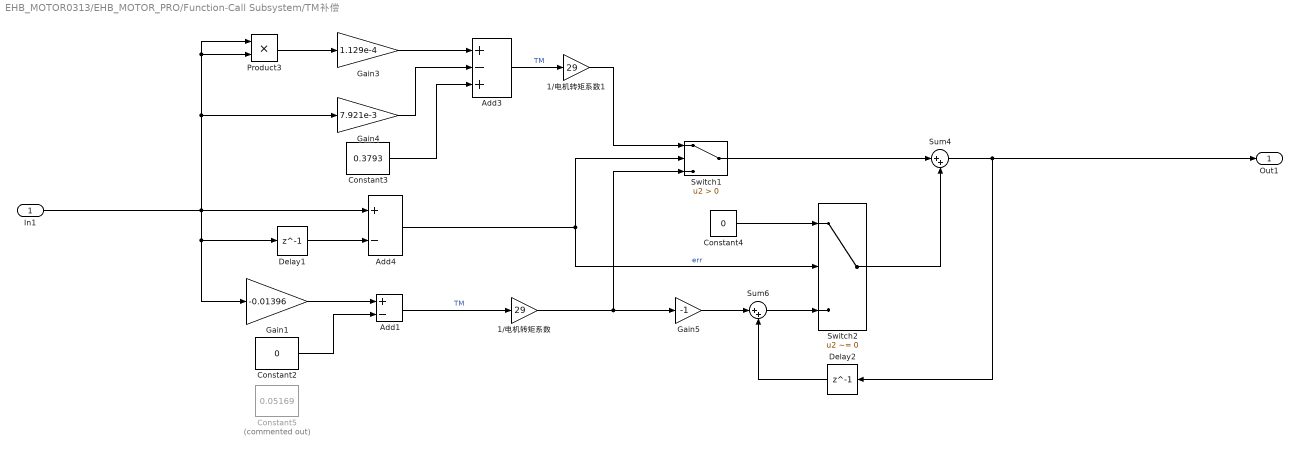
== system EHB_MOTOR0313/EHB_MOTOR_PRO/Function-Call Subsystem/TM补偿 ==
  In1 : Inport
  1/电机转矩系数 : Gain  Gain=29
  1/电机转矩系数1 : Gain  Gain=29
  Add1 : Sum  Inputs=+-
  Add3 : Sum  Inputs=+-+
  Add4 : Sum  Inputs=+-
  Constant2 : Constant  Value=0  OutDataTypeStr=single
  Constant3 : Constant  Value=0.3793  OutDataTypeStr=single
  Constant4 : Constant  Value=0  OutDataTypeStr=single
  Constant5 : Constant  Commented=on  Value=0.05169  OutDataTypeStr=single
  Delay1 : Delay  DelayLength=1
  Delay2 : Delay  DelayLength=1
  Gain1 : Gain  Gain=-0.01396
  Gain3 : Gain  Gain=1.129e-4
  Gain4 : Gain  Gain=7.921e-3
  Gain5 : Gain  Gain=-1
  Product3 : Product
  Sum4 : Sum  Inputs=|++
  Sum6 : Sum  Inputs=|++
  Switch1 : Switch  Criteria=u2 > Threshold  SaturateOnIntegerOverflow=off  InputSameDT=off
  Switch2 : Switch  Criteria=u2 ~= 0  SaturateOnIntegerOverflow=off  InputSameDT=off
  Out1 : Outport
  wires:
  Constant3/1 -> Add3/3
  1/电机转矩系数1/1 -> Switch1/1
  Gain5/1 -> Sum6/1
  Sum4/1 -> Delay2/1, Out1/1
  Sum6/1 -> Switch2/3
  Product3/1 -> Gain3/1
  Gain1/1 -> Add1/1
  Gain4/1 -> Add3/2
  Switch1/1 -> Sum4/1
  Switch2/1 -> Sum4/2
  Delay2/1 -> Sum6/2
  Constant4/1 -> Switch2/1
  In1/1 -> Product3/1, Product3/2, Gain4/1, Add4/1, Gain1/1, Delay1/1
  Delay1/1 -> Add4/2
  Constant2/1 -> Add1/2
  Add1/1 -> 1/电机转矩系数/1  "TM"
  Add3/1 -> 1/电机转矩系数1/1  "TM"
  Gain3/1 -> Add3/1
  Add4/1 -> Switch1/2, Switch2/2  "err"
  1/电机转矩系数/1 -> Gain5/1, Switch1/3

== system EHB_MOTOR0313/EHB_MOTOR_PRO/Function-Call Subsystem/pi2 ==
  In1 : Inport
  w_I : Inport  Port=2
  Delay : Delay  DelayLength=1
  Delay1 : Delay  DelayLength=1
  Gain : Gain  Gain=0.001
  Product : Product
  Saturation : Saturate  UpperLimit=0  LowerLimit=-1.57  OutDataTypeStr=single
  Sum : Sum  Inputs=|++
  Sum1 : Sum  Inputs=|++
  Sum2 : Sum  Inputs=|+-
  超前角 : Outport
  wires:
  Saturation/1 -> Sum2/1, 超前角/1
  w_I/1 -> Product/1
  Product/1 -> Gain/1
  Sum1/1 -> Delay1/1, Sum2/2, Saturation/1
  In1/1 -> Product/2
  Gain/1 -> Sum/1
  Sum/1 -> Sum1/1
  Delay1/1 -> Sum1/2
  Sum2/1 -> Delay/1
  Delay/1 -> Sum/2

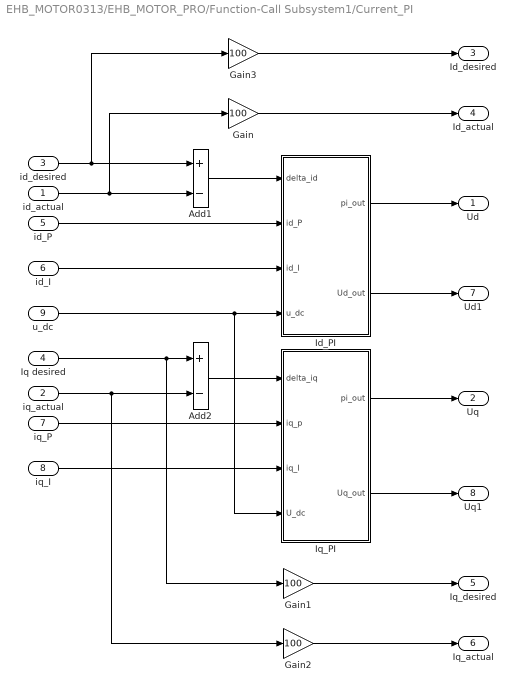
== system EHB_MOTOR0313/EHB_MOTOR_PRO/Function-Call Subsystem1/Current_PI ==
  id_actual : Inport  OutDataTypeStr=single
  iq_actual : Inport  Port=2  OutDataTypeStr=single
  id_desired : Inport  Port=3  OutDataTypeStr=single
  Iq desired : Inport  Port=4  OutDataTypeStr=single
  id_P : Inport  Port=5  OutDataTypeStr=single
  id_I : Inport  Port=6  OutDataTypeStr=single
  iq_P : Inport  Port=7  OutDataTypeStr=single
  iq_I : Inport  Port=8  OutDataTypeStr=single
  u_dc : Inport  Port=9
  Add1 : Sum  Inputs=+-  OutDataTypeStr=single
  Add2 : Sum  Inputs=+-  OutDataTypeStr=single
  Gain{,1..3} (4 alike) : Gain  Gain=100  OutDataTypeStr=int16
  Id_PI : Subsystem
  Iq_PI : Subsystem
  Ud : Outport  OutDataTypeStr=single  VectorParamsAs1DForOutWhenUnconnected=off
  Uq : Outport  Port=2  OutDataTypeStr=single  VectorParamsAs1DForOutWhenUnconnected=off
  Id_desired : Outport  Port=3  OutDataTypeStr=int16  VectorParamsAs1DForOutWhenUnconnected=off
  Id_actual : Outport  Port=4  OutDataTypeStr=int16  VectorParamsAs1DForOutWhenUnconnected=off
  Iq_desired : Outport  Port=5  OutDataTypeStr=int16  VectorParamsAs1DForOutWhenUnconnected=off
  Iq_actual : Outport  Port=6  OutDataTypeStr=int16  VectorParamsAs1DForOutWhenUnconnected=off
  Ud1 : Outport  Port=7  OutDataTypeStr=single  VectorParamsAs1DForOutWhenUnconnected=off
  Uq1 : Outport  Port=8  OutDataTypeStr=single  VectorParamsAs1DForOutWhenUnconnected=off
  wires:
  Add1/1 -> Id_PI/1(delta_id)
  id_desired/1 -> Gain3/1, Add1/1
  Add2/1 -> Iq_PI/1(delta_iq)
  Iq desired/1 -> Gain1/1, Add2/1
  iq_actual/1 -> Gain2/1, Add2/2
  id_actual/1 -> Gain/1, Add1/2
  Id_PI/1(pi_out) -> Ud/1
  Iq_PI/1(pi_out) -> Uq/1
  id_P/1 -> Id_PI/2(id_P)
  id_I/1 -> Id_PI/3(id_I)
  iq_P/1 -> Iq_PI/2(iq_p)
  iq_I/1 -> Iq_PI/3(iq_I)
  u_dc/1 -> Iq_PI/4(U_dc), Id_PI/4(u_dc)
  Gain/1 -> Id_actual/1
  Gain1/1 -> Iq_desired/1
  Gain2/1 -> Iq_actual/1
  Gain3/1 -> Id_desired/1
  Id_PI/2(Ud_out) -> Ud1/1
  Iq_PI/2(Uq_out) -> Uq1/1

== system EHB_MOTOR0313/EHB_MOTOR_PRO/Function-Call Subsystem1/Current_Transform ==
  sector : Inport
  iA : Inport  Port=2
  iB : Inport  Port=3
  IC : Inport  Port=4
  cos_theta : Inport  Port=5
  sin_theta : Inport  Port=6
  CLARK : Subsystem
  Ia_caculate : Subsystem
  Park : Subsystem
  d_current : Outport  OutDataTypeStr=single  VectorParamsAs1DForOutWhenUnconnected=off
  q_current : Outport  Port=2  OutDataTypeStr=single  VectorParamsAs1DForOutWhenUnconnected=off
  wires:
  iA/1 -> Ia_caculate/2(Ia_Inte)
  iB/1 -> Ia_caculate/3(Ib_Inte)
  CLARK/1(alpha_current) -> Park/1(alpha)
  CLARK/2(beta_current) -> Park/2(beta)
  cos_theta/1 -> Park/3(cos_theta)
  sin_theta/1 -> Park/4(sin_theta)
  Park/1(d_current) -> d_current/1
  Park/2(q_current) -> q_current/1
  IC/1 -> Ia_caculate/4(Ic_Inte)
  Ia_caculate/1(A) -> CLARK/1(IA)
  Ia_caculate/2(B) -> CLARK/2(IB)
  sector/1 -> Ia_caculate/1(sector)

== system EHB_MOTOR0313/EHB_MOTOR_PRO/Function-Call Subsystem1/Inverse_Park_Transform ==
  note: Inverse Park Transform
  Ud : Inport
  Uq : Inport  Port=2
  cos_theta : Inport  Port=3
  sin_theta : Inport  Port=4
  Add : Sum  OutDataTypeStr=single
  Add1 : Sum  Inputs=+-  OutDataTypeStr=single
  Product{,1..3} (4 alike) : Product  OutDataTypeStr=single  RndMeth=Zero
  alpha_voltage : Outport  VectorParamsAs1DForOutWhenUnconnected=off
  beta_voltage : Outport  Port=2  VectorParamsAs1DForOutWhenUnconnected=off
  wires:
  Product/1 -> Add/1
  Product1/1 -> Add/2
  Add/1 -> beta_voltage/1  "beta_voltage"
  Product2/1 -> Add1/1
  Product3/1 -> Add1/2
  Add1/1 -> alpha_voltage/1  "alpha_voltage"
  Ud/1 -> Product/1, Product2/1
  sin_theta/1 -> Product/2, Product3/2
  cos_theta/1 -> Product1/2, Product2/2
  Uq/1 -> Product1/1, Product3/1

== system EHB_MOTOR0313/EHB_MOTOR_PRO/Function-Call Subsystem1/PWM scaling ==
  PWM_Duty_Time : Inport
  Gain : Gain  Gain=7500  OutDataTypeStr=uint16
  Scope1 : Scope
  PWM_Numbers : Outport  VectorParamsAs1DForOutWhenUnconnected=off
  wires:
  PWM_Duty_Time/1 -> Gain/1
  Gain/1 -> Scope1/1, PWM_Numbers/1

== system EHB_MOTOR0313/EHB_MOTOR_PRO/Function-Call Subsystem1/SVPWM ==
  Ualfa : Inport  OutDataTypeStr=single
  Ubeta : Inport  Port=2
  Calculate_Phase_Voltages : Subsystem
  Sector Caculate : Subsystem
  sector : Outport  VectorParamsAs1DForOutWhenUnconnected=off
  phase_voltages : Outport  Port=2  VectorParamsAs1DForOutWhenUnconnected=off
  wires:
  Ualfa/1 -> Sector Caculate/1(alpha_voltage), Calculate_Phase_Voltages/2(Ualpha)
  Ubeta/1 -> Calculate_Phase_Voltages/3(Ubeta), Sector Caculate/2(beta_voltage)
  Sector Caculate/1(sector) -> sector/1, Calculate_Phase_Voltages/1(N)
  Calculate_Phase_Voltages/1(phase_voltages) -> phase_voltages/1

== system EHB_MOTOR0313/EHB_MOTOR_PRO/Function-Call Subsystem1/Subsystem ==
  In1 : Inport
  Gain1 : Gain  Gain=7.6699e-04  OutDataTypeStr=single
  n-D Lookup Table : Lookup_n-D  NumberOfTableDimensions=1  BreakpointsForDimension1=Sin_BreakPoint  BreakpointsForDimension3=[5, 7]  BreakpointsForDimension1DataTypeStr=Inherit: Inherit from 'Breakpoint data'  Table=Sin_Table  TableDataTypeStr=Inherit: Inherit from 'Table data'  ExtrapMethod=Clip  InternalRulePriority=Speed  OutDataTypeStr=Inherit: Inherit from 'Table data'  RndMeth=Simplest  InputSameDT=off
  n-D Lookup Table1 : Lookup_n-D  NumberOfTableDimensions=1  BreakpointsForDimension1=Sin_BreakPoint  BreakpointsForDimension3=[5, 7]  BreakpointsForDimension1DataTypeStr=Inherit: Inherit from 'Breakpoint data'  Table=Cos_Table  TableDataTypeStr=Inherit: Inherit from 'Table data'  ExtrapMethod=Clip  InternalRulePriority=Speed  OutDataTypeStr=Inherit: Inherit from 'Table data'  RndMeth=Simplest  InputSameDT=off
  cos : Outport  VectorParamsAs1DForOutWhenUnconnected=off
  Sin : Outport  Port=2  VectorParamsAs1DForOutWhenUnconnected=off
  wires:
  Gain1/1 -> n-D Lookup Table/1, n-D Lookup Table1/1
  In1/1 -> Gain1/1
  n-D Lookup Table/1 -> Sin/1
  n-D Lookup Table1/1 -> cos/1

== system EHB_MOTOR0313/EHB_MOTOR_PRO/Function-Call Subsystem1/electri_angle zero ==
  Theta_Inte : Inport
  Theta_zero : Inport  Port=2  OutDataTypeStr=uint16
  Angle_Val : Switch  Criteria=u2 ~= 0  Threshold=3032  OutDataTypeStr=uint16  SaturateOnIntegerOverflow=off  InputSameDT=off
  Constant : Constant  Value=8192  OutDataTypeStr=uint16
  Max_Count : Constant  Value=32768  OutDataTypeStr=uint16
  Mod : Math  Operator=mod  SignedPower=on
  Relational Operator : RelationalOperator  OutDataTypeStr=boolean  InputSameDT=off
  Theta_to_Max : Sum  Inputs=+-  OutDataTypeStr=uint16
  Zero_to_Theta : Sum  Inputs=++-  OutDataTypeStr=uint16
  Theta : Outport  VectorParamsAs1DForOutWhenUnconnected=off
  wires:
  Max_Count/1 -> Zero_to_Theta/1
  Theta_zero/1 -> Zero_to_Theta/3, Theta_to_Max/2, Relational Operator/2
  Theta_Inte/1 -> Zero_to_Theta/2, Theta_to_Max/1, Relational Operator/1
  Zero_to_Theta/1 -> Angle_Val/3
  Theta_to_Max/1 -> Angle_Val/1
  Relational Operator/1 -> Angle_Val/2
  Mod/1 -> Theta/1
  Angle_Val/1 -> Mod/1
  Constant/1 -> Mod/2

== system EHB_MOTOR0313/EHB_MOTOR_PRO/Function-Call Subsystem1/Current_PI/Id_PI ==
  delta_id : Inport  OutDataTypeStr=single
  id_P : Inport  Port=2  OutDataTypeStr=single
  id_I : Inport  Port=3  OutDataTypeStr=single
  u_dc : Inport  Port=4  OutDataTypeStr=single
  Delay : Delay  DelayLength=1
  Gain : Gain  Gain=1.732  OutDataTypeStr=single
  Id_sat : Saturate  UpperLimit=6.65  LowerLimit=-6.65  OutDataTypeStr=single
  Id_sat1 : Saturate  UpperLimit=6.65  LowerLimit=-6.65  OutDataTypeStr=single
  Id_sat2 : Saturate  UpperLimit=6.65  LowerLimit=-6.65  OutDataTypeStr=single
  Product : Product  OutDataTypeStr=single
  Product1 : Product  OutDataTypeStr=single
  Product2 : Product  OutDataTypeStr=single
  Sum : Sum  InputSameDT=on  OutDataTypeStr=single  SaturateOnIntegerOverflow=on
  Sum1 : Sum  Inputs=|++  OutDataTypeStr=single
  pi_out : Outport  OutDataTypeStr=single  VectorParamsAs1DForOutWhenUnconnected=off
  Ud_out : Outport  Port=2  OutDataTypeStr=single  VectorParamsAs1DForOutWhenUnconnected=off
  wires:
  delta_id/1 -> Product/1  "id_e"
  id_P/1 -> Product/2
  Product/1 -> Product1/1, Sum/1  "yp"
  id_I/1 -> Product1/2
  Id_sat/1 -> pi_out/1
  Id_sat1/1 -> Sum/2
  Sum1/1 -> Delay/1, Id_sat1/1
  Delay/1 -> Sum1/2
  Sum/1 -> Id_sat2/1
  Product2/1 -> Gain/1
  u_dc/1 -> Product2/2
  Gain/1 -> Id_sat/1
  Id_sat2/1 -> Ud_out/1, Product2/1
  Product1/1 -> Sum1/1

== system EHB_MOTOR0313/EHB_MOTOR_PRO/Function-Call Subsystem1/Current_PI/Iq_PI ==
  delta_iq : Inport  OutDataTypeStr=single
  iq_p : Inport  Port=2  OutDataTypeStr=single
  iq_I : Inport  Port=3  OutDataTypeStr=single
  U_dc : Inport  Port=4  OutDataTypeStr=single
  Delay : Delay  DelayLength=1
  Gain : Gain  Gain=1.732  OutDataTypeStr=single
  Iq_sat : Saturate  UpperLimit=6.65  LowerLimit=-6.65  OutDataTypeStr=single
  Iq_sat1 : Saturate  UpperLimit=6.65  LowerLimit=-6.65  OutDataTypeStr=single
  Iq_sat2 : Saturate  UpperLimit=6.65  LowerLimit=-6.65  OutDataTypeStr=single
  Product : Product  OutDataTypeStr=single
  Product1 : Product  OutDataTypeStr=single
  Product2 : Product
  Sum : Sum  InputSameDT=on  OutDataTypeStr=single  SaturateOnIntegerOverflow=on
  Sum1 : Sum  Inputs=|++  OutDataTypeStr=single
  pi_out : Outport  OutDataTypeStr=single  VectorParamsAs1DForOutWhenUnconnected=off
  Uq_out : Outport  Port=2  OutDataTypeStr=single  VectorParamsAs1DForOutWhenUnconnected=off
  wires:
  Product/1 -> Product1/1, Sum/1  "yp"
  delta_iq/1 -> Product/1  "iq_e"
  iq_p/1 -> Product/2  "iq_e"
  iq_I/1 -> Product1/2  "iq_e"
  Iq_sat/1 -> pi_out/1
  Iq_sat1/1 -> Sum/2
  Sum1/1 -> Delay/1, Iq_sat1/1
  Delay/1 -> Sum1/2
  Sum/1 -> Iq_sat2/1
  Product2/1 -> Gain/1
  U_dc/1 -> Product2/2
  Gain/1 -> Iq_sat/1
  Iq_sat2/1 -> Uq_out/1, Product2/1
  Product1/1 -> Sum1/1

== system EHB_MOTOR0313/EHB_MOTOR_PRO/Function-Call Subsystem1/Current_Transform/CLARK ==
  IA : Inport
  IB : Inport  Port=2
  Add : Sum  AccumDataTypeStr=single
  B_Gain : Gain  Gain=2  OutDataTypeStr=single
  Beta_Gain : Gain  Gain=0.5774  OutDataTypeStr=single
  alpha_current : Outport  OutDataTypeStr=single  VectorParamsAs1DForOutWhenUnconnected=off
  beta_current : Outport  Port=2  OutDataTypeStr=single  VectorParamsAs1DForOutWhenUnconnected=off
  wires:
  Add/1 -> Beta_Gain/1
  IB/1 -> B_Gain/1
  B_Gain/1 -> Add/2
  Beta_Gain/1 -> beta_current/1
  IA/1 -> alpha_current/1, Add/1

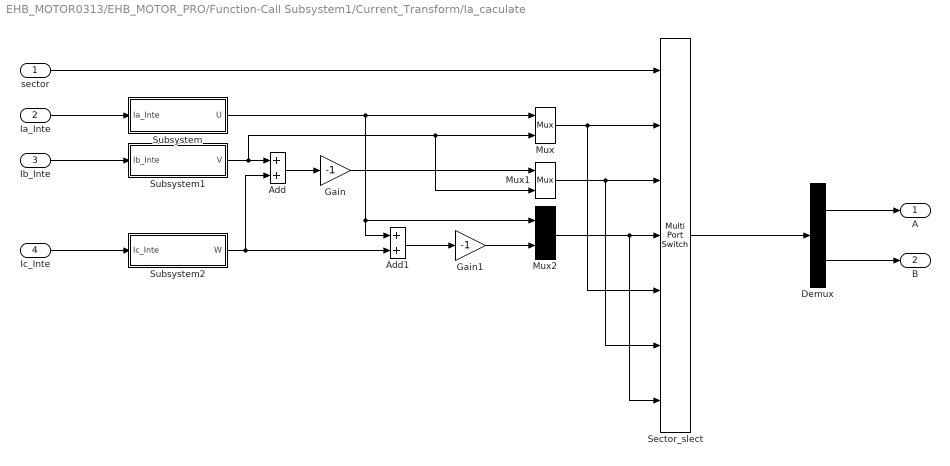
== system EHB_MOTOR0313/EHB_MOTOR_PRO/Function-Call Subsystem1/Current_Transform/Ia_caculate ==
  sector : Inport
  Ia_Inte : Inport  Port=2  OutDataTypeStr=uint16
  Ib_Inte : Inport  Port=3  OutDataTypeStr=uint16
  Ic_Inte : Inport  Port=4  OutDataTypeStr=uint16
  Add : Sum
  Add1 : Sum
  Demux : Demux  Outputs=2
      settings: DisplayOption=none
  Gain : Gain  Gain=-1
  Gain1 : Gain  Gain=-1
  Mux : Mux  Inputs=2
  Mux1 : Mux  Inputs=2
  Mux2 : Mux  Inputs=2
  Sector_slect : MultiPortSwitch  Inputs=6  DiagnosticForDefault=None  OutDataTypeStr=single  SaturateOnIntegerOverflow=off  InputSameDT=off
  Subsystem : Subsystem
  Subsystem1 : Subsystem
  Subsystem2 : Subsystem
  A : Outport
  B : Outport  Port=2
  wires:
  Ia_Inte/1 -> Subsystem/1(Ia_Inte)
  Subsystem/1(U) -> Mux/1, Add1/1, Mux2/1
  Ib_Inte/1 -> Subsystem1/1(Ib_Inte)
  Subsystem1/1(V) -> Add/1, Mux1/2, Mux/2
  Ic_Inte/1 -> Subsystem2/1(Ic_Inte)
  Subsystem2/1(W) -> Add1/2, Add/2
  Add/1 -> Gain/1
  Gain/1 -> Mux1/1
  Add1/1 -> Gain1/1
  Gain1/1 -> Mux2/2
  Mux/1 -> Sector_slect/2, Sector_slect/5
  Mux1/1 -> Sector_slect/6, Sector_slect/3
  Mux2/1 -> Sector_slect/7, Sector_slect/4
  Sector_slect/1 -> Demux/1
  Demux/1 -> A/1
  Demux/2 -> B/1
  sector/1 -> Sector_slect/1

== system EHB_MOTOR0313/EHB_MOTOR_PRO/Function-Call Subsystem1/Current_Transform/Park ==
  note: Converts balanced two-phase orthogonal stationary system to an orthogonal rotating reference frame.
  note: Park Transform
  alpha : Inport
  beta : Inport  Port=2
  cos_theta : Inport  Port=3
  sin_theta : Inport  Port=4
  Add : Sum  Inputs=-+  OutDataTypeStr=single
  Add1 : Sum  OutDataTypeStr=single
  Product{,1..3} (4 alike) : Product  OutDataTypeStr=single  RndMeth=Zero
  Scope : Scope
  d_current : Outport  OutDataTypeStr=single  VectorParamsAs1DForOutWhenUnconnected=off
  q_current : Outport  Port=2  OutDataTypeStr=single  VectorParamsAs1DForOutWhenUnconnected=off
  wires:
  beta/1 -> Product3/1, Product1/1
  Add1/1 -> d_current/1  "d_current"
  alpha/1 -> Product/1, Product2/1
  Product1/1 -> Scope/1, Add/2
  cos_theta/1 -> Product1/2, Product2/2
  Product3/1 -> Add1/2
  Product2/1 -> Add1/1
  sin_theta/1 -> Product3/2, Product/2
  Product/1 -> Add/1
  Add/1 -> q_current/1  "q_current"

== system EHB_MOTOR0313/EHB_MOTOR_PRO/Function-Call Subsystem1/SVPWM/Calculate_Phase_Voltages ==
  N : Inport  OutDataTypeStr=uint8
  Ualpha : Inport  Port=2  OutDataTypeStr=single
  Ubeta : Inport  Port=3  OutDataTypeStr=single
  Bus Creator : BusCreator  Inputs=3
  Bus_Voltage : Constant  OutDataTypeStr=single
  Phase_Voltage_Sectors_1_and_4 : Subsystem
  Sector_slect : MultiPortSwitch  Inputs=6  DiagnosticForDefault=None  OutDataTypeStr=single  SaturateOnIntegerOverflow=off  InputSameDT=off
  U_Sectors_2_and_5 : Subsystem
  U_Sectors_3_and_6 : Subsystem
  phase_voltages : Outport  VectorParamsAs1DForOutWhenUnconnected=off
  wires:
  Ualpha/1 -> Bus Creator/2  "U_alpha"
  Ubeta/1 -> Bus Creator/3  "U_beta"
  Bus_Voltage/1 -> Bus Creator/1  "Bus_Voltage"
  N/1 -> Sector_slect/1
  Bus Creator/1 -> U_Sectors_3_and_6/1(Bus_Beta), Phase_Voltage_Sectors_1_and_4/1(Bus_Alpha_Beta), U_Sectors_2_and_5/1(Bus_Alpha)
  Sector_slect/1 -> phase_voltages/1
  U_Sectors_3_and_6/1(UVW_Sector_3_and_6) -> Sector_slect/4, Sector_slect/7
  Phase_Voltage_Sectors_1_and_4/1(UVW_Sector_1_and_4) -> Sector_slect/2, Sector_slect/5
  U_Sectors_2_and_5/1(UVW_Sector_2_and_5) -> Sector_slect/6, Sector_slect/3

== system EHB_MOTOR0313/EHB_MOTOR_PRO/Function-Call Subsystem1/SVPWM/Sector Caculate ==
  note: Phase Advanced Inverse Clarke Transform
  note: Projects the quadrature (beta) component (as opposed to the conventional inverse Clarke transform
      | which projects the alpha component).
  alpha_voltage : Inport
  beta_voltage : Inport  Port=2
  Add : Sum  Inputs=-+
  Add1 : Sum  Inputs=--
  Calculate_Phase_Advanced_Sector : Sum  Inputs=+++  AccumDataTypeStr=uint8  OutDataTypeStr=uint8
  Compare_VA_To_Zero : simulink/Logic and Bit Operations/Compare To Zero  relop=>  OutDataTypeStr=uint8
  Compare_VB_To_Zero : simulink/Logic and Bit Operations/Compare To Zero  relop=>  OutDataTypeStr=uint8
  Compare_VC_To_Zero : simulink/Logic and Bit Operations/Compare To Zero  relop=>  OutDataTypeStr=uint8
  Gain : Gain  Gain=0.5  OutDataTypeStr=Inherit: Same as input
  Gain1 : Gain  Gain=0.866  OutDataTypeStr=Inherit: Same as input
  Sector_Gain_VB : Gain  Gain=2  ParamDataTypeStr=int16  OutDataTypeStr=uint8
  Sector_Gain_VC : Gain  Gain=4  ParamDataTypeStr=int16  OutDataTypeStr=uint8
  Sector_Lookup_Table : LookupNDDirect  NumberOfTableDimensions=1  Table=[2,2,6,1,4,3,5]  TableDataTypeStr=uint8
      settings: AttributesFormatString=-------------------------------\nTable: %<Table>
  sector : Outport  VectorParamsAs1DForOutWhenUnconnected=off
  wires:
  Sector_Gain_VC/1 -> Calculate_Phase_Advanced_Sector/3
  alpha_voltage/1 -> Gain1/1
  Calculate_Phase_Advanced_Sector/1 -> Sector_Lookup_Table/1
  Sector_Lookup_Table/1 -> sector/1
  Compare_VA_To_Zero/1 -> Calculate_Phase_Advanced_Sector/1
  beta_voltage/1 -> Compare_VA_To_Zero/1, Gain/1
  Add1/1 -> Compare_VC_To_Zero/1  "voltage_phase_c"
  Compare_VC_To_Zero/1 -> Sector_Gain_VC/1
  Compare_VB_To_Zero/1 -> Sector_Gain_VB/1
  Sector_Gain_VB/1 -> Calculate_Phase_Advanced_Sector/2
  Gain1/1 -> Add1/2, Add/2
  Gain/1 -> Add1/1, Add/1
  Add/1 -> Compare_VB_To_Zero/1  "voltage_phase_b"

== system EHB_MOTOR0313/EHB_MOTOR_PRO/Function-Call Subsystem1/Current_Transform/Ia_caculate/Subsystem ==
  Ia_Inte : Inport  OutDataTypeStr=uint16
  Add : Sum  Inputs=+-  OutDataTypeStr=int16
  Constant2 : Constant  Value=2039  OutDataTypeStr=int16
  Gain1 : Gain  Gain=0.0814  OutDataTypeStr=single
  U : Outport
  wires:
  Gain1/1 -> U/1
  Ia_Inte/1 -> Add/1
  Constant2/1 -> Add/2
  Add/1 -> Gain1/1
